simulink model "analog_mod"  (Simulink 7.6)
settings: Solver=FixedStepDiscrete  StartTime=0.0  StopTime=100  FixedStep=1  RelTol=1e-3
libraries: simulink x24
settings Model: Creator=jordan  LastModifiedBy=jordan
settings DataIOCC: LimitDataPoints=off  SaveOutput=off  SignalLogging=off  DSMLogging=off  SaveTime=off
settings OptimizationCC: BlockReduction=off  ConditionallyExecuteInputs=off

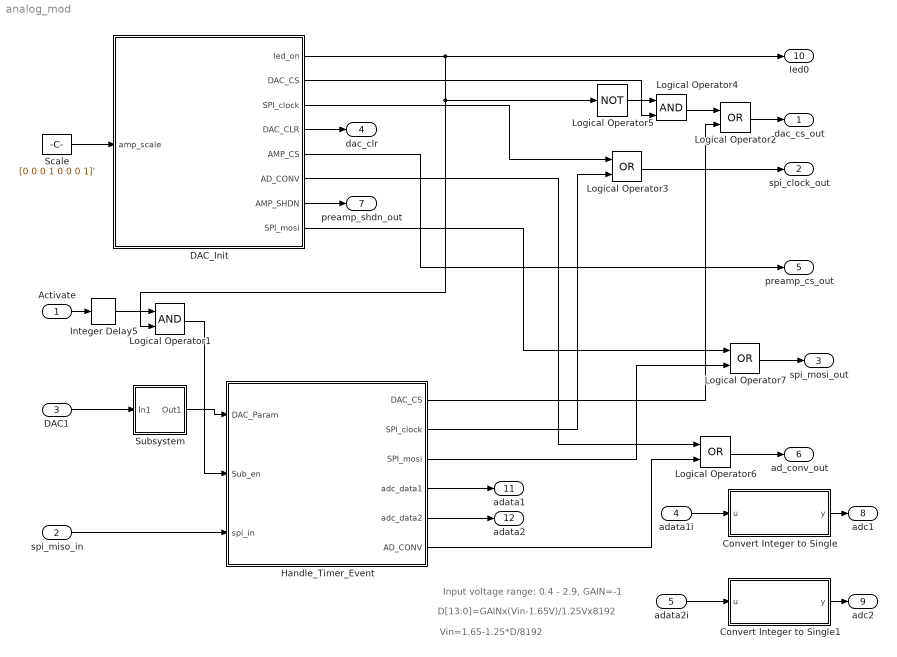
== system analog_mod ==
  note: Input voltage range: 0.4 - 2.9, GAIN=-1
  note: D[13:0]=GAINx(Vin-1.65V)/1.25Vx8192
  note: Vin=1.65-1.25*D/8192
  Activate : Inport  OutDataTypeStr=boolean
  spi_miso_in : Inport  Port=2  OutDataTypeStr=boolean
  DAC1 : Inport  Port=3  OutDataTypeStr=fixdt(1,12,0)
  adata1i : Inport  Port=4  OutDataTypeStr=fixdt(1,14,0)
  adata2i : Inport  Port=5  OutDataTypeStr=fixdt(1,14,0)
  Convert Integer to Single : Stateflow chart  TreatAsAtomicUnit=on
  Convert Integer to Single1 : Stateflow chart  TreatAsAtomicUnit=on
  DAC_Init : Stateflow chart  TreatAsAtomicUnit=on
  Handle_Timer_Event : Stateflow chart  TreatAsAtomicUnit=on
  Integer Delay5 : simulink/Discrete/Integer Delay  NumDelays=1  vinit=0.0  samptime=-1
  Logical Operator1 : Logic  AllPortsSameDT=off  OutDataTypeStr=boolean
  Logical Operator{2..3,6..7} (4 alike) : Logic  Operator=OR  AllPortsSameDT=off  OutDataTypeStr=boolean
  Logical Operator4 : Logic  AllPortsSameDT=off  OutDataTypeStr=boolean
  Logical Operator5 : Logic  Operator=NOT  AllPortsSameDT=off  OutDataTypeStr=boolean
  Scale : Constant  Value=[0 0 0 1 0 0 0 1]'  OutDataTypeStr=boolean
  Subsystem : Subsystem
  dac_cs_out : Outport
  spi_clock_out : Outport  Port=2
  spi_mosi_out : Outport  Port=3
  dac_clr : Outport  Port=4
  preamp_cs_out : Outport  Port=5
  ad_conv_out : Outport  Port=6
  preamp_shdn_out : Outport  Port=7
  adc1 : Outport  Port=8  OutDataTypeStr=uint32
  adc2 : Outport  Port=9  OutDataTypeStr=uint32
  led0 : Outport  Port=10
  adata1 : Outport  Port=11  OutDataTypeStr=boolean  PortDimensions=14
  adata2 : Outport  Port=12  OutDataTypeStr=boolean  PortDimensions=14
  wires:
  Activate/1 -> Integer Delay5/1
  Subsystem/1(Out1) -> Handle_Timer_Event/1(DAC_Param)
  DAC_Init/1(led_on) -> Logical Operator1/2, Logical Operator5/1, led0/1
  Logical Operator1/1 -> Handle_Timer_Event/2(Sub_en)
  Logical Operator2/1 -> dac_cs_out/1
  DAC_Init/2(DAC_CS) -> Logical Operator4/2
  Logical Operator3/1 -> spi_clock_out/1
  DAC_Init/3(SPI_clock) -> Logical Operator3/1
  Handle_Timer_Event/3(SPI_mosi) -> Logical Operator7/2
  DAC_Init/4(DAC_CLR) -> dac_clr/1
  Logical Operator4/1 -> Logical Operator2/1
  Logical Operator5/1 -> Logical Operator4/1
  DAC_Init/5(AMP_CS) -> preamp_cs_out/1
  DAC_Init/6(AD_CONV) -> Logical Operator6/1
  spi_miso_in/1 -> Handle_Timer_Event/3(spi_in)
  DAC_Init/7(AMP_SHDN) -> preamp_shdn_out/1
  Logical Operator6/1 -> ad_conv_out/1
  Handle_Timer_Event/6(AD_CONV) -> Logical Operator6/2
  adata1i/1 -> Convert Integer to Single/1(u)
  adata2i/1 -> Convert Integer to Single1/1(u)
  DAC1/1 -> Subsystem/1(In1)
  Handle_Timer_Event/1(DAC_CS) -> Logical Operator2/2
  Handle_Timer_Event/2(SPI_clock) -> Logical Operator3/2
  Integer Delay5/1 -> Logical Operator1/1
  Scale/1 -> DAC_Init/1(amp_scale)
  DAC_Init/8(SPI_mosi) -> Logical Operator7/1
  Logical Operator7/1 -> spi_mosi_out/1
  Convert Integer to Single/1(y) -> adc1/1
  Convert Integer to Single1/1(y) -> adc2/1
  Handle_Timer_Event/4(adc_data1) -> adata1/1
  Handle_Timer_Event/5(adc_data2) -> adata2/1

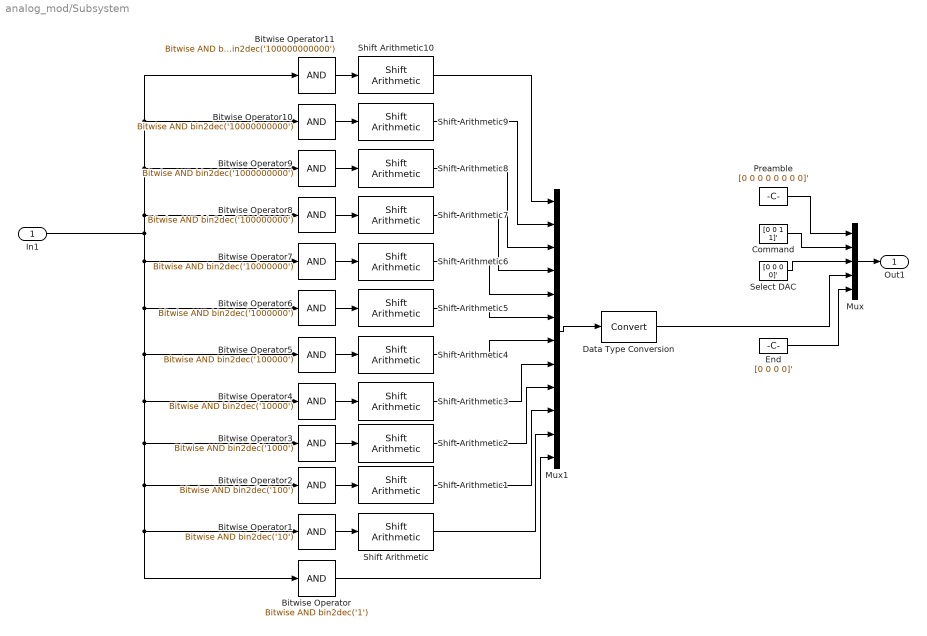
== system analog_mod/Subsystem ==
  In1 : Inport  OutDataTypeStr=fixdt(1,12,0)
  Bitwise Operator : simulink/Logic and Bit Operations/Bitwise Operator  logicop=AND  UseBitMask=on  BitMask=bin2dec('1')  BitMaskRealWorld=Stored Integer
  Bitwise Operator1 : simulink/Logic and Bit Operations/Bitwise Operator  logicop=AND  UseBitMask=on  BitMask=bin2dec('10')  BitMaskRealWorld=Stored Integer
  Bitwise Operator10 : simulink/Logic and Bit Operations/Bitwise Operator  logicop=AND  UseBitMask=on  BitMask=bin2dec('10000000000')  BitMaskRealWorld=Stored Integer
  Bitwise Operator11 : simulink/Logic and Bit Operations/Bitwise Operator  logicop=AND  UseBitMask=on  BitMask=bin2dec('100000000000')  BitMaskRealWorld=Stored Integer
  Bitwise Operator2 : simulink/Logic and Bit Operations/Bitwise Operator  logicop=AND  UseBitMask=on  BitMask=bin2dec('100')  BitMaskRealWorld=Stored Integer
  Bitwise Operator3 : simulink/Logic and Bit Operations/Bitwise Operator  logicop=AND  UseBitMask=on  BitMask=bin2dec('1000')  BitMaskRealWorld=Stored Integer
  Bitwise Operator4 : simulink/Logic and Bit Operations/Bitwise Operator  logicop=AND  UseBitMask=on  BitMask=bin2dec('10000')  BitMaskRealWorld=Stored Integer
  Bitwise Operator5 : simulink/Logic and Bit Operations/Bitwise Operator  logicop=AND  UseBitMask=on  BitMask=bin2dec('100000')  BitMaskRealWorld=Stored Integer
  Bitwise Operator6 : simulink/Logic and Bit Operations/Bitwise Operator  logicop=AND  UseBitMask=on  BitMask=bin2dec('1000000')  BitMaskRealWorld=Stored Integer
  Bitwise Operator7 : simulink/Logic and Bit Operations/Bitwise Operator  logicop=AND  UseBitMask=on  BitMask=bin2dec('10000000')  BitMaskRealWorld=Stored Integer
  Bitwise Operator8 : simulink/Logic and Bit Operations/Bitwise Operator  logicop=AND  UseBitMask=on  BitMask=bin2dec('100000000')  BitMaskRealWorld=Stored Integer
  Bitwise Operator9 : simulink/Logic and Bit Operations/Bitwise Operator  logicop=AND  UseBitMask=on  BitMask=bin2dec('1000000000')  BitMaskRealWorld=Stored Integer
  Command : Constant  Value=[0 0 1 1]'  OutDataTypeStr=boolean
  Data Type Conversion : DataTypeConversion
  End : Constant  Value=[0 0 0 0]'  OutDataTypeStr=boolean
  Mux : Mux  Inputs=5
  Mux1 : Mux  Inputs=12
  Preamble : Constant  Value=[0 0 0 0 0 0 0 0]'  OutDataTypeStr=boolean
  Select DAC : Constant  Value=[0 0 0 0]'  OutDataTypeStr=boolean
  Shift Arithmetic : simulink/Logic and Bit Operations/Shift Arithmetic  SystemSampleTime=-1  nBitShiftRight=1  nBinPtShiftRight=0
  Shift Arithmetic1 : simulink/Logic and Bit Operations/Shift Arithmetic  SystemSampleTime=-1  nBitShiftRight=2  nBinPtShiftRight=0
  Shift Arithmetic10 : simulink/Logic and Bit Operations/Shift Arithmetic  SystemSampleTime=-1  nBitShiftRight=11  nBinPtShiftRight=0
  Shift Arithmetic2 : simulink/Logic and Bit Operations/Shift Arithmetic  SystemSampleTime=-1  nBitShiftRight=3  nBinPtShiftRight=0
  Shift Arithmetic3 : simulink/Logic and Bit Operations/Shift Arithmetic  SystemSampleTime=-1  nBitShiftRight=4  nBinPtShiftRight=0
  Shift Arithmetic4 : simulink/Logic and Bit Operations/Shift Arithmetic  SystemSampleTime=-1  nBitShiftRight=5  nBinPtShiftRight=0
  Shift Arithmetic5 : simulink/Logic and Bit Operations/Shift Arithmetic  SystemSampleTime=-1  nBitShiftRight=6  nBinPtShiftRight=0
  Shift Arithmetic6 : simulink/Logic and Bit Operations/Shift Arithmetic  SystemSampleTime=-1  nBitShiftRight=7  nBinPtShiftRight=0
  Shift Arithmetic7 : simulink/Logic and Bit Operations/Shift Arithmetic  SystemSampleTime=-1  nBitShiftRight=8  nBinPtShiftRight=0
  Shift Arithmetic8 : simulink/Logic and Bit Operations/Shift Arithmetic  SystemSampleTime=-1  nBitShiftRight=9  nBinPtShiftRight=0
  Shift Arithmetic9 : simulink/Logic and Bit Operations/Shift Arithmetic  SystemSampleTime=-1  nBitShiftRight=10  nBinPtShiftRight=0
  Out1 : Outport
  wires:
  Preamble/1 -> Mux/1
  Command/1 -> Mux/2
  Select DAC/1 -> Mux/3
  End/1 -> Mux/5
  Mux/1 -> Out1/1
  In1/1 -> Bitwise Operator11/1, Bitwise Operator10/1, Bitwise Operator9/1, Bitwise Operator8/1, Bitwise Operator7/1, Bitwise Operator6/1, Bitwise Operator5/1, Bitwise Operator4/1, Bitwise Operator3/1, Bitwise Operator2/1, Bitwise Operator/1, Bitwise Operator1/1
  Bitwise Operator1/1 -> Shift Arithmetic/1
  Bitwise Operator2/1 -> Shift Arithmetic1/1
  Bitwise Operator3/1 -> Shift Arithmetic2/1
  Bitwise Operator4/1 -> Shift Arithmetic3/1
  Bitwise Operator5/1 -> Shift Arithmetic4/1
  Bitwise Operator6/1 -> Shift Arithmetic5/1
  Bitwise Operator7/1 -> Shift Arithmetic6/1
  Bitwise Operator8/1 -> Shift Arithmetic7/1
  Bitwise Operator9/1 -> Shift Arithmetic8/1
  Bitwise Operator10/1 -> Shift Arithmetic9/1
  Bitwise Operator11/1 -> Shift Arithmetic10/1
  Bitwise Operator/1 -> Mux1/12
  Shift Arithmetic/1 -> Mux1/11
  Shift Arithmetic1/1 -> Mux1/10
  Shift Arithmetic2/1 -> Mux1/9
  Shift Arithmetic3/1 -> Mux1/8
  Shift Arithmetic4/1 -> Mux1/7
  Shift Arithmetic5/1 -> Mux1/6
  Shift Arithmetic6/1 -> Mux1/5
  Shift Arithmetic7/1 -> Mux1/4
  Shift Arithmetic8/1 -> Mux1/3
  Shift Arithmetic9/1 -> Mux1/2
  Shift Arithmetic10/1 -> Mux1/1
  Mux1/1 -> Data Type Conversion/1
  Data Type Conversion/1 -> Mux/4

== matlab function Convert Integer to Single ==
  data: u input fixdt(1,14,0); y output uint32
function y = fcn(u)
%#eml

sig=uint8(0);
exp=uint8(0);
frac=fi(0,0,23,0);

%Transform two's complement integer into unnormalized
%single number
buf=fi(0,1,14,0);
if (u>0)
    sig=uint8(0);
    buf=u;
    frac1=fi(buf,0,23,0);
else
    sig=uint8(1);
    buf=-u;
    frac1=fi(buf,0,23,0);
end

%Normalize floating-point number
buf1=fi(frac1,0,24,0);
p=fi(0,0,5,0);
mask=fi(2^22,0,24,0);
for ind=1:23
    c=bitand(buf1,mask);
    if (c==0)
        buf1=bitshift(buf1,1);
        p=fi(p+1,0,5,0);
    end
end
p=fi(p+1,0,5,0);
buf1=bitshift(fi(frac1,0,24,0),uint8(p));
mask1=fi(2^23-1,0,24,0);
buf1=bitand(buf1,mask1);
frac=fi(buf1,0,23,0);
exp=uint8(127+(22-p));

%Compose floating-point number
z=uint32(0);
if sig
    z=uint32(bitshift(uint32(1),31));
end
buf2=uint32(bitshift(uint32(exp),23));
z=bitor(z,buf2);
z=bitor(z,uint32(frac));
y=z;

== stateflow chart DAC_Init ==
  settings: executeAtInitialization=1
  state DAC_init
  state Led_is_Off
  state Wait6
  state Wait3
  state Wait7
  state Wait8
  state Wait9
  state AMP_Init
  state AMP_Init1
  state Wait1
  state Wait10
  state Wait11
  state Wait12
  state Wait13
  state End_Init
  state Wait14
  state Wait15
  state Wait16
  (default) -> Led_is_Off
  Led_is_Off -> DAC_init : [led_on==0]{SPI_clock=0;
      | DAC_CS=1;
      | DAC_CLR=1;
      | AMP_CS=1; AMP_SHDN=0;/*AMP_SHDN=1;*/
      | AD_CONV=0;
      | ind1=0;}
  Wait6 -> AMP_Init : {DAC_CLR=1;
      | /*led_on=1;*/}
  Wait7 -> (junction 28)
  (junction 29) -> Wait3 : {ind1++;}
  (junction 28) -> (junction 29) [order 1] : [ind1<255]
  (junction 28) -> Wait6 [order 2] : {DAC_CLR=0;}
  DAC_init -> (junction 28)
  Wait3 -> Wait9
  Wait9 -> Wait8
  Wait8 -> Wait7
  End_Init -> Led_is_Off
  AMP_Init -> AMP_Init1 : {ind1=0;
      | AMP_CS=0;
      | SPI_mosi=amp_scale[0];}
  AMP_Init1 -> Wait1
  Wait1 -> Wait10
  Wait10 -> Wait11 : {SPI_clock=1;
      | ind1++;}
  Wait11 -> Wait12
  Wait12 -> Wait13
  (junction 30) -> AMP_Init1 [order 1] : [ind1<8]{
      | SPI_mosi=amp_scale[ind1];}
  Wait13 -> (junction 30) : {SPI_clock=0;}
  Wait16 -> End_Init : {AMP_CS=1;
      | SPI_mosi=0;
      | led_on=1;}
  (junction 30) -> Wait14 [order 2]
  Wait14 -> Wait15
  Wait15 -> Wait16
  data: led_on output boolean; DAC_CS output boolean =1; SPI_clock output boolean =0; DAC_CLR output boolean =1; ind1 local uint8; AMP_CS output boolean; AD_CONV output boolean; AMP_SHDN output boolean; amp_scale input boolean size=8; SPI_mosi output boolean

== stateflow chart Handle_Timer_Event ==
  settings: executeAtInitialization=1
  state Led_is_On
  state Led_is_Off
  state Wait11
  state Wait1
  state Wait3
  state Wait7
  state Wait12
  state AD_Start
  state Wait9
  state Wait10
  state Wait17
  state Wait14
  state Wait15
  state Wait18
  state Wait19
  state Wait20
  state Wait21
  state Wait22
  state Wait23
  state Wait24
  state Wait25
  (default) -> Led_is_Off
  Led_is_Off -> Led_is_On : [Sub_en==1]{
      | DAC_CS=0;
      | ind1=0;}
  Wait1 -> Wait7 : {SPI_clock=1;}
  Wait3 -> (junction 88)
  Wait7 -> Wait3 : {ind1++;
      | SPI_clock=0;}
  (junction 88) -> (junction 89) [order 1] : [ind1<32]
  (junction 89) -> Wait1 : {SPI_mosi=DAC_Param[ind1];}
  Led_is_On -> (junction 88)
  (junction 88) -> AD_Start [order 2] : {DAC_CS=1;}
  (junction 90) -> (junction 92) [order 2] : {SPI_clock=1;
      | ind1=0;}
  Wait17 -> Wait11 : {SPI_clock=1;}
  AD_Start -> Wait9 : {AD_CONV=1;}
  Wait9 -> Wait10 : {AD_CONV=0;
      | ind1=0;}
  Wait10 -> Wait17
  Wait15 -> Wait12 : {SPI_clock=0;
      | ind1++;}
  Wait14 -> (junction 90)
  Wait11 -> Wait15
  Wait12 -> Wait14 : [ind1>1]{
      | adc_data1[ind1-2]=spi_in;}
  (junction 90) -> Wait11 [order 1] : [ind1<15]{SPI_clock=1;}
  Wait21 -> Wait19 : {SPI_clock=0;
      | ind1++;}
  Wait20 -> (junction 91)
  Wait19 -> Wait20 : [ind1>1]{
      | adc_data2[ind1-2]=spi_in;}
  (junction 91) -> Wait18 [order 1] : [ind1<15]{SPI_clock=1;}
  Wait18 -> Wait21
  Wait25 -> Led_is_Off
  (junction 91) -> Wait22 [order 2] : {SPI_clock=1;}
  Wait22 -> Wait23 : {SPI_clock=0;}
  Wait23 -> Wait24 : {SPI_clock=1;}
  Wait24 -> Wait25 : {SPI_clock=0;}
  (junction 92) -> Wait18
  data: DAC_CS output boolean =1; SPI_clock output boolean =0; SPI_mosi output boolean; DAC_Param input boolean size=32; ind1 local uint8; Sub_en input boolean; adc_data1 output boolean size=14; adc_data2 output boolean size=14; spi_in input boolean; AD_CONV output boolean

== matlab function Convert Integer to Single1 ==
  data: u input fixdt(1,14,0); y output uint32
function y = fcn(u)
%#eml

sig=uint8(0);
exp=uint8(0);
frac=fi(0,0,23,0);

%Transform two's complement integer into unnormalized
%single number
buf=fi(0,1,14,0);
if (u>0)
    sig=uint8(0);
    buf=u;
    frac1=fi(buf,0,23,0);
else
    sig=uint8(1);
    buf=-u;
    frac1=fi(buf,0,23,0);
end

%Normalize floating-point number
buf1=fi(frac1,0,24,0);
p=fi(0,0,5,0);
mask=fi(2^22,0,24,0);
for ind=1:23
    c=bitand(buf1,mask);
    if (c==0)
        buf1=bitshift(buf1,1);
        p=fi(p+1,0,5,0);
    end
end
p=fi(p+1,0,5,0);
buf1=bitshift(fi(frac1,0,24,0),uint8(p));
mask1=fi(2^23-1,0,24,0);
buf1=bitand(buf1,mask1);
frac=fi(buf1,0,23,0);
exp=uint8(127+(22-p));

%Compose floating-point number
z=uint32(0);
if sig
    z=uint32(bitshift(uint32(1),31));
end
buf2=uint32(bitshift(uint32(exp),23));
z=bitor(z,buf2);
z=bitor(z,uint32(frac));
y=z;
